simulink model "SAC_simulink"  (R2025b)
settings: Solver=ode4  StartTime=0.0  StopTime=180  FixedStep=0.01  RelTol=1e-3
values from neighbouring files (symbols this model uses):
  action_limits_lower = 0.88    [main_SAC.m]
  action_limits_upper = 1.07    [main_SAC.m]
  b0 = (1-t)^3    [ph7_teta_vincolato_new.m]
  k = Num_k./(Den_k + 1e-6)    [ph7_teta_vincolato_new.m]
  par_phys = struct    [main_SAC.m]    (also in test_all_agents_random_training_domain.m)
  rigeneration_step_s = 300    [main_SAC.m]
  T = resultsTable(ok, :)    [test_all_agents_random_training_domain.m]
  target = [0; 0; 0]    [test_all_agents_random_training_domain.m]
  Ts = 150    [main_SAC.m]    (also in test_all_agents_random_training_domain.m)
undefined symbols (not defined in the file or in its folder): delay, delta_a_max, h_max, h_min, k0_target, k1_target, k_L, max_idx, mean_vertical_velocity, meters_end_zf, r_max, r_min, s_f_time, t1_max_rad, t1_min_rad, t_step, wc, X0, yaw_max, yaw_min
libraries: slctrl_adaptive x3, aerolibobsolete x1, aerolibasang x1, simulink x1, aerolibatmos2 x1, rllib x1
(part 1 of 2)
settings Model: PauseTimes=0.01  PacingRate=0.200000  Creator=massy  LastModifiedBy=nicom
settings DebuggingCC: UnconnectedInputMsg=warning  UnconnectedOutputMsg=warning  UnconnectedLineMsg=warning
settings ModelReferenceCC: EnableRefExpFcnMdlSchedulingChecks=on
settings RTWCC: GPUComputeCapability=3.5  DLArmComputeVersion=19.05

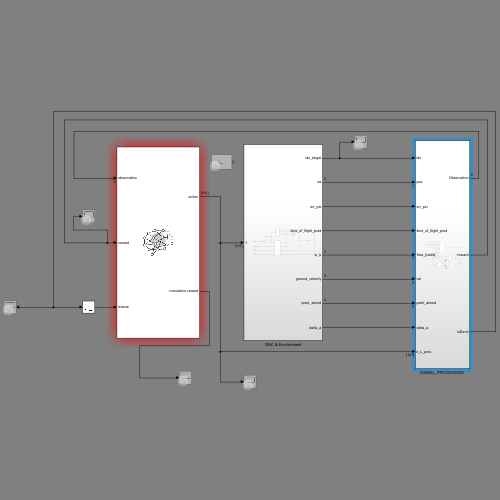
[thumbnail: Simulink's stored preview of the top-level diagram]
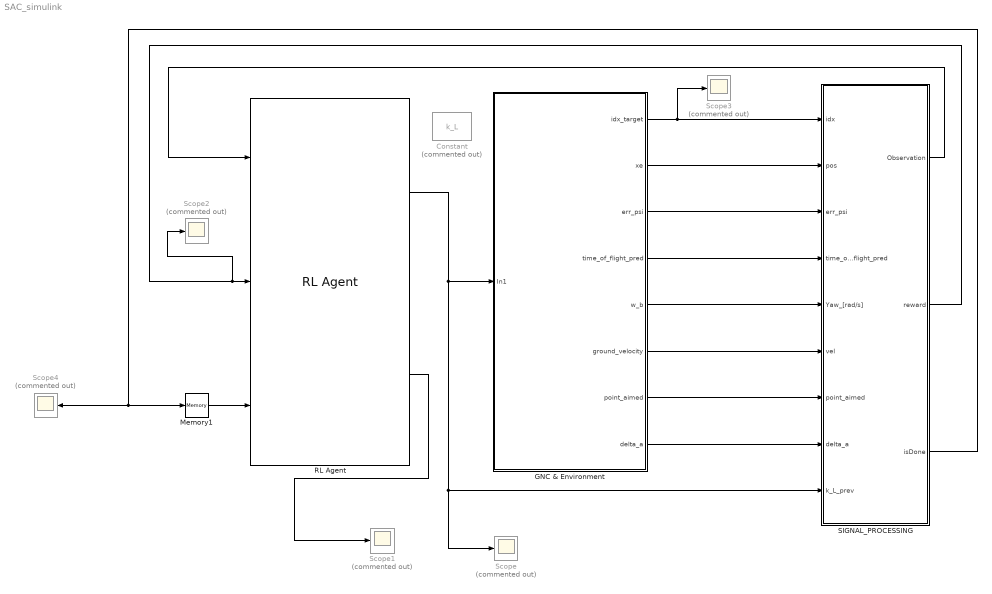
== system SAC_simulink ==
  Constant : Constant  Commented=on  Value=k_L
  GNC & Environment : Subsystem
  Memory1 : Memory
  RL Agent : rllib/RL Agent  Agent=agent  ExternalActionAsInput=off  ProvideLastAction=off  ProvideCumRwd=on  TreatAsDirectFeedthrough=on  UseStrictObservationDataTypes=off
  "SIGNAL_PROCESSING " : Subsystem
  Scope{,1..4} (5 alike) : Scope  Commented=on
      Scope settings: ActiveDisplayYMinimum=0.48959660530090332  ActiveDisplayYMaximum=2.4895966053009033  DataLoggingVariableName=ScopeData29
      Scope1 settings: ActiveDisplayYMinimum=-18280.567213697534  ActiveDisplayYMaximum=2455.6337548888514  DataLoggingVariableName=ScopeData35
      Scope2 settings: ActiveDisplayYMinimum=-16245.428943711315  ActiveDisplayYMaximum=-3791.1395065981656  DataLoggingVariableName=ScopeData36
      Scope3 settings: ActiveDisplayYMinimum=-22.849241680887388  ActiveDisplayYMaximum=119.97274269411264  DataLoggingVariableName=ScopeData37
      Scope4 settings: ActiveDisplayYMinimum=-0.12499999999999997  ActiveDisplayYMaximum=1.125  DataLoggingVariableName=ScopeData14
  wires:
  "SIGNAL_PROCESSING "/1(Observation) -> RL Agent/1
  GNC & Environment/1(idx_target) -> Scope3/1, "SIGNAL_PROCESSING "/1(idx)
  GNC & Environment/3(err_psi) -> "SIGNAL_PROCESSING "/3(err_psi)
  GNC & Environment/2(xe) -> "SIGNAL_PROCESSING "/2(pos)
  Memory1/1 -> RL Agent/3
  RL Agent/1 -> Scope/1, "SIGNAL_PROCESSING "/9(k_L_prev), GNC & Environment/1(In1)
  GNC & Environment/8(delta_a) -> "SIGNAL_PROCESSING "/8(delta_a)
  GNC & Environment/6(ground_velocity) -> "SIGNAL_PROCESSING "/6(vel)
  GNC & Environment/4(time_of_flight_pred) -> "SIGNAL_PROCESSING "/4(time_of_flight_pred)
  GNC & Environment/7(point_aimed) -> "SIGNAL_PROCESSING "/7(point_aimed)
  GNC & Environment/5(w_b) -> "SIGNAL_PROCESSING "/5(Yaw_[rad/s])
  "SIGNAL_PROCESSING "/3(isDone) -> Scope4/1, Memory1/1
  RL Agent/2 -> Scope1/1
  "SIGNAL_PROCESSING "/2(reward) -> Scope2/1, RL Agent/2

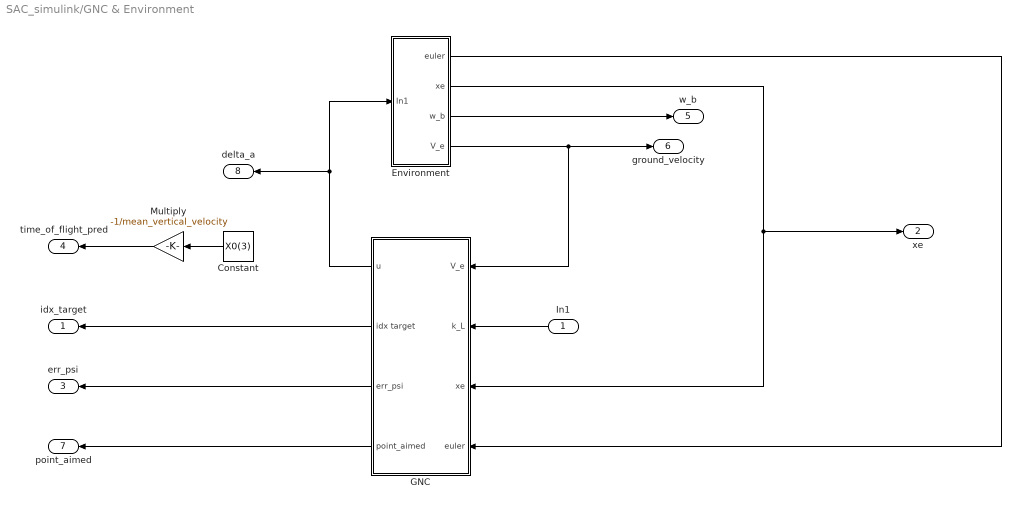
== system SAC_simulink/GNC & Environment ==
  In1 : Inport
  Constant : Constant  Value=X0(3)
  Environment : Subsystem
  GNC : Subsystem
  Multiply : Gain  Gain=-1/mean_vertical_velocity
  idx_target : Outport
  xe : Outport  Port=2
  err_psi : Outport  Port=3
  time_of_flight_pred : Outport  Port=4
  w_b : Outport  Port=5
  ground_velocity : Outport  Port=6
  point_aimed : Outport  Port=7
  delta_a : Outport  Port=8
  wires:
  Multiply/1 -> time_of_flight_pred/1
  GNC/3(err_psi) -> err_psi/1
  Environment/3(w_b) -> w_b/1
  Environment/1(euler) -> GNC/4(euler)
  Environment/2(xe) -> GNC/3(xe), xe/1
  GNC/2(idx target) -> idx_target/1
  GNC/1(u) -> delta_a/1, Environment/1(In1)
  Environment/4(V_e) -> ground_velocity/1, GNC/1(V_e)
  GNC/4(point_aimed) -> point_aimed/1
  Constant/1 -> Multiply/1
  In1/1 -> GNC/2(k_L)

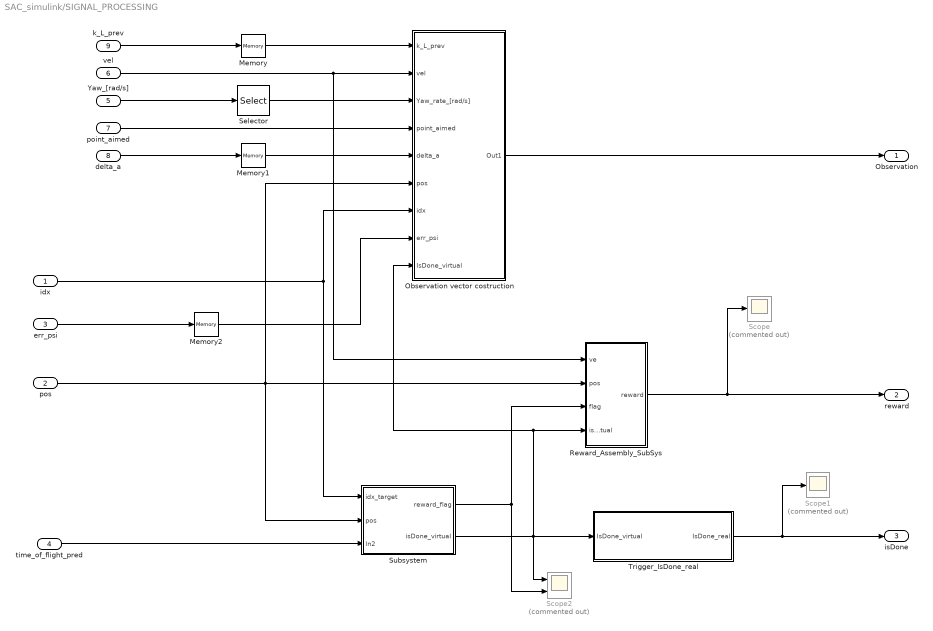
== system SAC_simulink/SIGNAL_PROCESSING  ==
  idx : Inport
  pos : Inport  Port=2
  err_psi : Inport  Port=3
  time_of_flight_pred : Inport  Port=4
  Yaw_[rad/s] : Inport  Port=5
  vel : Inport  Port=6
  point_aimed : Inport  Port=7
  delta_a : Inport  Port=8
  k_L_prev : Inport  Port=9
  Memory : Memory
  Memory1 : Memory
  Memory2 : Memory
  Observation vector costruction : Subsystem
  Reward_Assembly_SubSys : Subsystem
  Scope : Scope  Commented=on
      settings: ActiveDisplayYMinimum=-21750  ActiveDisplayYMaximum=-14250
  Scope1 : Scope  Commented=on
      settings: ActiveDisplayYMinimum=-0.72691328594836357  ActiveDisplayYMaximum=2.2813607561654949  DataLoggingVariableName=ScopeData17
  Scope2 : Scope  Commented=on  NumInputPorts=2
      settings: ActiveDisplayYMinimum=-0.13410064239828712  ActiveDisplayYMaximum=1.3815578158458244  DataLoggingVariableName=ScopeData18
  Selector : Selector  InputPortWidth=3  IndexOptions=Index vector (dialog)  Indices=[ 3]  OutputSizes=1
  Subsystem : Subsystem
  Trigger_IsDone_real : Subsystem
  Observation : Outport
  reward : Outport  Port=2
  isDone : Outport  Port=3
  wires:
  Subsystem/1(reward_flag) -> Scope2/2, Reward_Assembly_SubSys/3(flag)
  idx/1 -> Observation vector costruction/7(idx), Subsystem/1(idx_target)
  err_psi/1 -> Memory2/1
  point_aimed/1 -> Observation vector costruction/4(point_aimed)
  Subsystem/2(isDone_virtual) -> Scope2/1, Trigger_IsDone_real/1(IsDone_virtual), Reward_Assembly_SubSys/4(isDone_virtual), Observation vector costruction/9(IsDone_virtual)
  pos/1 -> Subsystem/2(pos), Reward_Assembly_SubSys/2(pos), Observation vector costruction/6(pos)
  Reward_Assembly_SubSys/1(reward) -> Scope/1, reward/1
  Yaw_[rad/s]/1 -> Selector/1
  time_of_flight_pred/1 -> Subsystem/3(In2)
  Observation vector costruction/1(Out1) -> Observation/1
  delta_a/1 -> Memory1/1
  Selector/1 -> Observation vector costruction/3(Yaw_rate_[rad/s])
  Trigger_IsDone_real/1(IsDone_real) -> Scope1/1, isDone/1
  k_L_prev/1 -> Memory/1
  vel/1 -> Reward_Assembly_SubSys/1(ve), Observation vector costruction/2(vel)
  Memory1/1 -> Observation vector costruction/5(delta_a)
  Memory2/1 -> Observation vector costruction/8(err_psi)
  Memory/1 -> Observation vector costruction/1(k_L_prev)

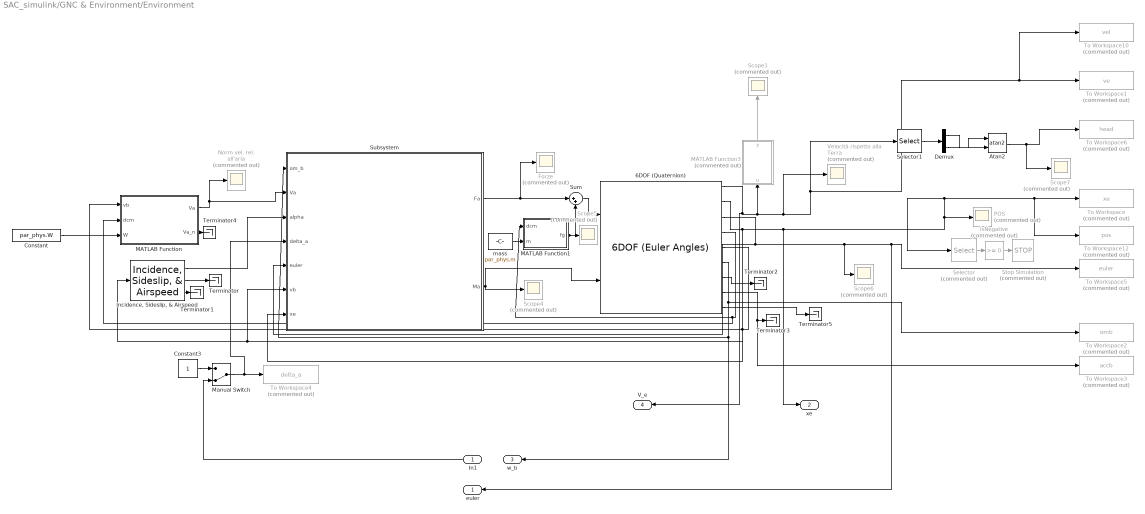
== system SAC_simulink/GNC & Environment/Environment ==
  In1 : Inport
  6DOF (Quaternion) : aerolibobsolete/6DOF (Euler Angles)  units=Metric (MKS)  mtype=Fixed  rep=Quaternion  xme_0=X0  Vm_0=V0  eul_0=euler  pm_0=w0  mass_0=par_phys.m  mass_e=0.5  mass_f=2.0  inertia=par_phys.I  inertia_e=eye(3)  inertia_f=2*eye(3)  k_quat=1.0  vre_flag=on  abi_flag=on  aMode=0  xme_statename=''  Vm_statename=''  eul_statename=''  quat_statename=''  pm_statename=''  mass_statename=''
  Atan2 : Trigonometry  Operator=atan2
  Constant : Constant  Value=par_phys.W
  Constant3 : Constant
  Demux : Demux  Outputs=2
  Forze : Scope  Commented=on
      settings: ActiveDisplayYMinimum=-111.7562  ActiveDisplayYMaximum=149.47198  DataLoggingVariableName=ScopeData4
  "Incidence, Sideslip, & Airspeed" : aerolibasang/Incidence, Sideslip, & Airspeed
  IsNegative : simulink/Logic and Bit Operations/Compare To Zero  Commented=on  relop=>=  OutDataTypeStr=boolean
      settings: LibrarySourceBlock=|
      | simulink/Quick Insert/Logic and Bit
      | Operations/IsNegative
  MATLAB Function : MATLAB Function  TreatAsAtomicUnit=on
  MATLAB Function1 : MATLAB Function  TreatAsAtomicUnit=on
  MATLAB Function3 : MATLAB Function  Commented=on  TreatAsAtomicUnit=on
  Manual Switch : ManualSwitch  CurrentSetting=0
  Norm vel. rel. all'aria : Scope  Commented=on
      settings: ActiveDisplayYMinimum=8.90491  ActiveDisplayYMaximum=12.9997  DataLoggingVariableName=ScopeData3
  POS : Scope  Commented=on
      settings: ActiveDisplayYMinimum=-1583.3551657510689  ActiveDisplayYMaximum=8026.0269716415532
  Scope{1,4..7} (5 alike) : Scope  Commented=on
      Scope1 settings: ActiveDisplayYMinimum=-1  ActiveDisplayYMaximum=1
      Scope4 settings: ActiveDisplayYMinimum=-1.26764  ActiveDisplayYMaximum=1.42182  DataLoggingVariableName=ScopeData5
      Scope5 settings: ActiveDisplayYMinimum=-38.15496  ActiveDisplayYMaximum=51.10944  DataLoggingVariableName=ScopeData6
      Scope6 settings: ActiveDisplayYMinimum=-1  ActiveDisplayYMaximum=1
      Scope7 settings: ActiveDisplayYMinimum=-1  ActiveDisplayYMaximum=1
  Selector : Selector  Commented=on  InputPortWidth=3  IndexOptions=Index vector (dialog)  Indices=[3]  OutputSizes=1
  Selector1 : Selector  InputPortWidth=3  IndexOptions=Index vector (dialog)  Indices=[1 2]  OutputSizes=1
  Stop Simulation : Stop  Commented=on
  Subsystem : Subsystem
  Sum : Sum  Inputs=|++
  Terminator{,1..5} (6 alike) : Terminator
  To Workspace : ToWorkspace  Commented=on  VariableName=xe  SampleTime=-1
  To Workspace1 : ToWorkspace  Commented=on  VariableName=ve  SampleTime=-1
  To Workspace10 : ToWorkspace  Commented=on  VariableName=vel  SaveFormat=Timeseries  SampleTime=-1
  To Workspace12 : ToWorkspace  Commented=on  VariableName=pos  SaveFormat=Timeseries  SampleTime=-1
  To Workspace2 : ToWorkspace  Commented=on  VariableName=omb  SampleTime=-1
  To Workspace3 : ToWorkspace  Commented=on  VariableName=accb  SampleTime=-1
  To Workspace4 : ToWorkspace  Commented=on  VariableName=delta_a  SampleTime=-1
  To Workspace5 : ToWorkspace  Commented=on  VariableName=euler  SampleTime=-1
  To Workspace6 : ToWorkspace  Commented=on  VariableName=head  SampleTime=-1
  Velocità rispetto alla Terra : Scope  Commented=on
      settings: ActiveDisplayYMinimum=-13.738515568500244  ActiveDisplayYMaximum=14.244609911524053  DataLoggingVariableName=ScopeData2
  mass : Constant  Value=par_phys.m
  euler : Outport
  xe : Outport  Port=2
  w_b : Outport  Port=3
  V_e : Outport  Port=4
  wires:
  Constant/1 -> MATLAB Function/3(W)
  Subsystem/2(Ma) -> Scope4/1, 6DOF (Quaternion)/2
  MATLAB Function1/1(fg) -> Sum/2, Scope5/1
  MATLAB Function/1(Va) -> Norm vel. rel. all'aria/1, Subsystem/2(Va)
  Constant3/1 -> Manual Switch/1
  6DOF (Quaternion)/3 -> Subsystem/5(euler), euler/1, To Workspace5/1, Scope6/1
  Atan2/1 -> Scope7/1, To Workspace6/1
  6DOF (Quaternion)/7 -> Terminator2/1
  Selector1/1 -> Demux/1
  Subsystem/1(Fa) -> Forze/1, Sum/1
  6DOF (Quaternion)/6 -> To Workspace2/1, w_b/1, Subsystem/1(om_b)
  MATLAB Function3/1(y) -> Scope1/1
  6DOF (Quaternion)/2 -> xe/1, Selector/1, To Workspace12/1, To Workspace/1, POS/1, Subsystem/7(xe)
  6DOF (Quaternion)/4 -> MATLAB Function1/1(dcm), MATLAB Function/2(dcm)
  6DOF (Quaternion)/5 -> "Incidence, Sideslip, & Airspeed"/1, Subsystem/6(vb), MATLAB Function/1(vb)
  In1/1 -> Manual Switch/2
  6DOF (Quaternion)/8 -> To Workspace3/1, Terminator3/1
  "Incidence, Sideslip, & Airspeed"/2 -> Terminator/1
  Sum/1 -> 6DOF (Quaternion)/1
  Demux/2 -> Atan2/1
  Demux/1 -> Atan2/2
  "Incidence, Sideslip, & Airspeed"/1 -> Subsystem/3(alpha)
  "Incidence, Sideslip, & Airspeed"/3 -> Terminator1/1
  Manual Switch/1 -> Subsystem/4(delta_a), To Workspace4/1
  mass/1 -> MATLAB Function1/2(m)
  MATLAB Function/2(Va_n) -> Terminator4/1
  6DOF (Quaternion)/1 -> V_e/1, Selector1/1, To Workspace10/1, To Workspace1/1, Velocità rispetto alla Terra/1, MATLAB Function3/1(u)
  Selector/1 -> IsNegative/1
  IsNegative/1 -> Stop Simulation/1
  6DOF (Quaternion)/9 -> Terminator5/1

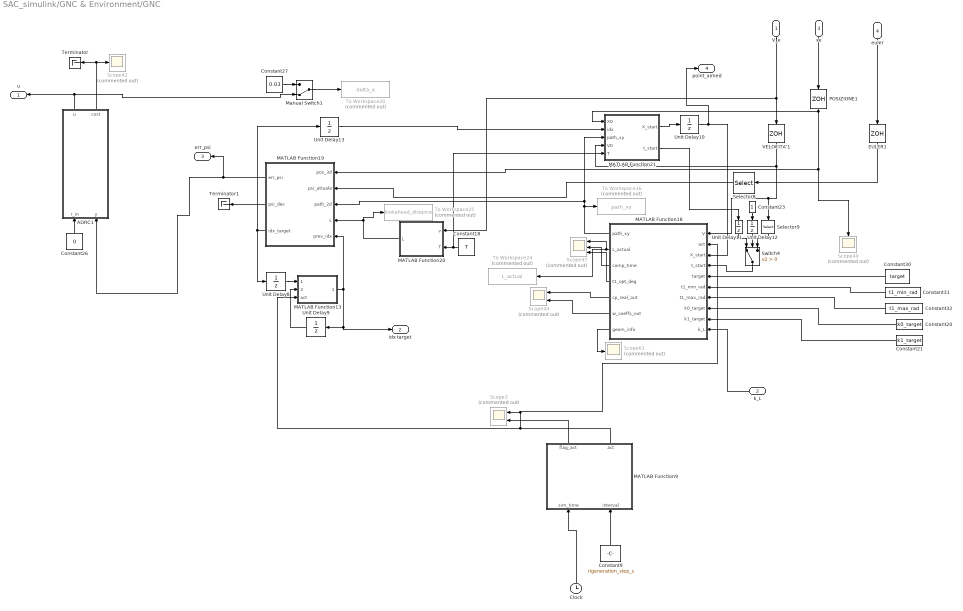
== system SAC_simulink/GNC & Environment/GNC ==
  V_e : Inport
  k_L : Inport  Port=2
  xe : Inport  Port=3
  euler : Inport  Port=4
  ADRC1 : Subsystem  mask{b0=-b0, wc=wc, wo=k*wc, Ts=t_step, x0=0, sat_u=0.03, sat_l=-0.03, rate_u=0.006, rate_l=-0.006}
      mask prompts: b0 "Critical Gain b0"; wc "Controller Bandwidth (rad/sec)"; wo "Observer Bandwidth (rad/sec)"; Ts "Sample Time"; x0 "Initial Condition"; sat_u "Upper bound"; sat_l "Lower bound"; rate_u "Upper bound"; rate_l "Lower bound"
      mask init:
      | % --- Codice di Inizializzazione Maschera ADRC ---
      | 
      | % 1. Calcolo dei parametri ESO
      | % (Mappa la bandwidth 'wo' nel dominio discreto Z)
      | beta = exp(-wo * Ts);
      | 
      | % 2. Guadagni Luenberger (vettore L)
      | % Formule per posizionare i 3 poli dell'osservatore in 'beta'
      | l1 = 1 - beta^3;
      | l2 = (3*(1-beta)^2 * (1+beta)) / (2*Ts);
      | l3 = (1-beta)^3 / (Ts^2);
      | 
      | % Vettore che i Gain interni si aspettano
      | ld = [l1; l2; l3]; 
      | 
      | % 3. Matrice Sistema Discreto (Ad)
      | % Modello doppio integratore (posizione, velocità, disturbo)
      | ad = [1, Ts, Ts^2/2;
      |       0,  1,    Ts;
      |       0,  0,     1];
      | 
      | % 4. Matrice Ingresso Discreto (Bd)
      | bd = [b0 * Ts^2/2;
      |       b0 * Ts;
      |       0];
      | 
      | % 5. Matrice Uscita (C)
      | c = [1 0 0];
      mask DialogControl DescTextVar Prompt: Parameters ADRC
      mask DialogControl Saturation Prompt: Saturation
      mask DialogControl Container4 Prompt: Rate Limiter
  Clock : Clock
  Constant18 : Constant  Value=T
  Constant20 : Constant  Value=k0_target
  Constant21 : Constant  Value=k1_target
  Constant23 : Constant
  Constant26 : Constant  Value=0
  Constant27 : Constant  Value=0.03
  Constant30 : Constant  Value=target
  Constant31 : Constant  Value=t1_min_rad
  Constant32 : Constant  Value=t1_max_rad
  Constant9 : Constant  Value=rigeneration_step_s
  EULER1 : ZeroOrderHold  SampleTime=-1
  MATLAB Function13 : MATLAB Function  TreatAsAtomicUnit=on
  MATLAB Function18 : MATLAB Function  TreatAsAtomicUnit=on
  MATLAB Function19 : MATLAB Function  TreatAsAtomicUnit=on
  MATLAB Function20 : MATLAB Function  TreatAsAtomicUnit=on
  MATLAB Function21 : MATLAB Function  TreatAsAtomicUnit=on
  MATLAB Function9 : MATLAB Function  TreatAsAtomicUnit=on
  Manual Switch1 : ManualSwitch  CurrentSetting=0
  POSIZIONE1 : ZeroOrderHold  SampleTime=-1
  Scope3 : Scope  Commented=on  NumInputPorts=2
      settings: ActiveDisplayYMinimum=-1.25  ActiveDisplayYMaximum=1.25  DataLoggingVariableName=ScopeData8
  Scope40 : Scope  Commented=on
      settings: ActiveDisplayYMinimum=-341.60221967749681  ActiveDisplayYMaximum=750.13712237085417  DataLoggingVariableName=ScopeData73
  Scope42 : Scope  Commented=on
      settings: ActiveDisplayYMinimum=-1  ActiveDisplayYMaximum=1  DataLoggingVariableName=ScopeData75
  Scope44 : Scope  Commented=on  NumInputPorts=2
      settings: ActiveDisplayYMinimum=-745.73859428255776  ActiveDisplayYMaximum=1354.574191363215  DataLoggingVariableName=ScopeData77
  Scope47 : Scope  Commented=on  NumInputPorts=3
      settings: ActiveDisplayYMinimum=-1672.2830379019078  ActiveDisplayYMaximum=3185.7011907738192  DataLoggingVariableName=ScopeData80
  Scope61 : Scope  Commented=on
      settings: DataLoggingVariableName=ScopeData94
  Selector8 : Selector  InputPortWidth=3  IndexOptions=Index vector (dialog)  Indices=3  OutputSizes=1
  Selector9 : Selector  InputPortWidth=3  IndexOptions=Index vector (dialog)  Indices=[1 2]  OutputSizes=1
  Switch4 : Switch  Criteria=u2 > Threshold  SaturateOnIntegerOverflow=off  InputSameDT=off
  Terminator : Terminator
  Terminator1 : Terminator
  To Workspace16 : ToWorkspace  Commented=on  VariableName=path_xy  SaveFormat=Timeseries  SampleTime=-1
  To Workspace20 : ToWorkspace  Commented=on  VariableName=delta_a  SampleTime=-1
  To Workspace24 : ToWorkspace  Commented=on  VariableName=L_actual  SaveFormat=Timeseries  SampleTime=-1
  To Workspace25 : ToWorkspace  Commented=on  VariableName=lookahead_distance  SaveFormat=Timeseries  SampleTime=-1
  Unit Delay10 : UnitDelay  InitialCondition=X0  SampleTime=-1  HasFrameUpgradeWarning=on
  Unit Delay11 : UnitDelay  InitialCondition=[0;0]  SampleTime=-1  HasFrameUpgradeWarning=on
  Unit Delay12 : UnitDelay  InitialCondition=[0;0]  SampleTime=-1  HasFrameUpgradeWarning=on
  Unit Delay13 : UnitDelay  InitialCondition=1  SampleTime=-1  HasFrameUpgradeWarning=on
  Unit Delay8 : UnitDelay  InitialCondition=1  SampleTime=-1  HasFrameUpgradeWarning=on
  Unit Delay9 : UnitDelay  InitialCondition=1  SampleTime=-1  HasFrameUpgradeWarning=on
  VELOCITA'1 : ZeroOrderHold  SampleTime=-1
  u : Outport
  idx target : Outport  Port=2
  err_psi : Outport  Port=3
  point_aimed : Outport  Port=4
  wires:
  MATLAB Function18/7(geom_info) -> Scope61/1
  Unit Delay8/1 -> MATLAB Function13/1(prev_idx)
  MATLAB Function18/2(L_actual) -> To Workspace24/1, Scope47/1
  MATLAB Function18/6(w_coeffs_out) -> Scope44/2
  Constant27/1 -> Manual Switch1/1
  Switch4/1 -> MATLAB Function18/4(t_start)
  MATLAB Function20/1(L) -> To Workspace25/1, MATLAB Function19/4(L)
  Unit Delay12/1 -> Switch4/2
  Manual Switch1/1 -> To Workspace20/1
  MATLAB Function21/1(X_start) -> Unit Delay10/1
  Unit Delay13/1 -> MATLAB Function21/2(idx)
  MATLAB Function18/1(path_xy) -> To Workspace16/1, MATLAB Function21/3(path_xy), MATLAB Function19/3(path_2d)
  Selector9/1 -> Switch4/3
  Constant20/1 -> MATLAB Function18/8(k0_target)
  Constant31/1 -> MATLAB Function18/6(t1_min_rad)
  MATLAB Function18/4(t1_opt_deg) -> Scope47/3
  MATLAB Function21/2(t_start) -> Unit Delay11/1
  Constant21/1 -> MATLAB Function18/9(k1_target)
  Constant26/1 -> ADRC1/1(r_in)
  POSIZIONE1/1 -> Scope40/1, MATLAB Function19/1(pos_3d), MATLAB Function21/1(X0)
  MATLAB Function19/1(err_psi) -> ADRC1/2(y), err_psi/1
  Unit Delay9/1 -> MATLAB Function13/2(old_idx)
  Unit Delay11/1 -> Switch4/1
  Constant32/1 -> MATLAB Function18/7(t1_max_rad)
  MATLAB Function13/1(prev_idx_clean) -> idx target/1, Unit Delay9/1, MATLAB Function19/5(prev_idx)
  MATLAB Function19/3(idx_target) -> Unit Delay13/1, Unit Delay8/1
  MATLAB Function18/3(comp_time) -> Scope47/2
  MATLAB Function18/5(cp_real_out) -> Scope44/1
  Constant23/1 -> Unit Delay12/1
  ADRC1/2(cost) -> Terminator/1, Scope42/1
  Selector8/1 -> MATLAB Function19/2(psi_attuale)
  EULER1/1 -> Selector8/1
  VELOCITA'1/1 -> MATLAB Function18/1(V), Selector9/1, MATLAB Function21/4(V0)
  Constant18/1 -> MATLAB Function21/5(T), MATLAB Function20/2(T)
  Constant30/1 -> MATLAB Function18/5(target)
  Unit Delay10/1 -> point_aimed/1, MATLAB Function18/3(X_start)
  ADRC1/1(u) -> Manual Switch1/2, u/1
  k_L/1 -> MATLAB Function18/10(k_L)
  euler/1 -> EULER1/1
  xe/1 -> POSIZIONE1/1
  V_e/1 -> VELOCITA'1/1, MATLAB Function20/1(v)
  MATLAB Function9/2(act) -> MATLAB Function13/3(act), MATLAB Function18/2(act), Scope3/1
  Clock/1 -> MATLAB Function9/1(sim_time)
  MATLAB Function9/1(flag_act) -> Scope3/2
  Constant9/1 -> MATLAB Function9/2(interval)
  MATLAB Function19/2(psi_des) -> Terminator1/1

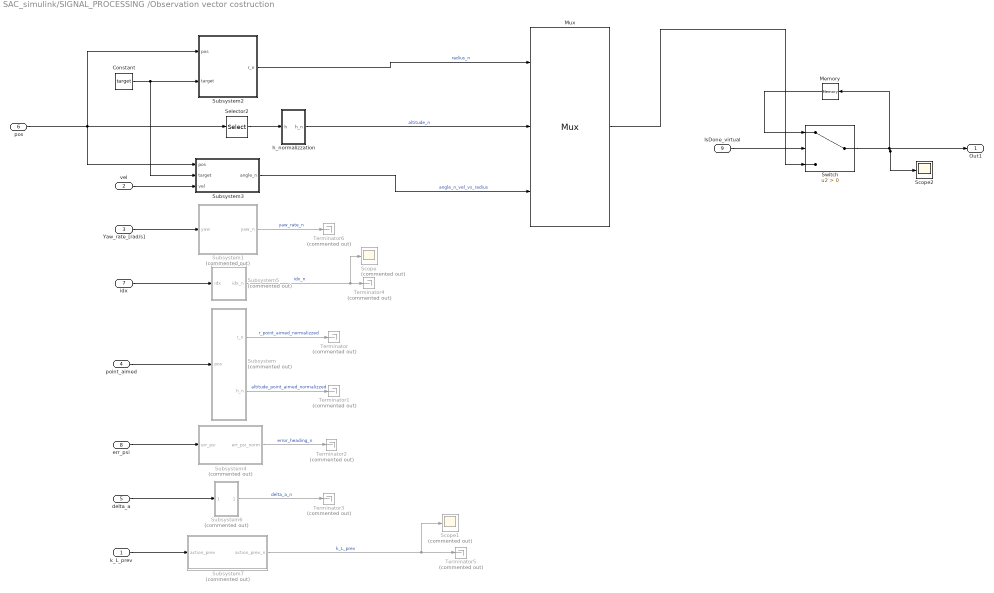
== system SAC_simulink/SIGNAL_PROCESSING /Observation vector costruction ==
  k_L_prev : Inport
  vel : Inport  Port=2
  Yaw_rate_[rad/s] : Inport  Port=3
  point_aimed : Inport  Port=4
  delta_a : Inport  Port=5
  pos : Inport  Port=6
  idx : Inport  Port=7
  err_psi : Inport  Port=8
  IsDone_virtual : Inport  Port=9
  Constant : Constant  Value=target
  Memory : Memory
  Mux : Mux  Inputs=3
  Scope : Scope  Commented=on
      settings: ActiveDisplayYMinimum=-1  ActiveDisplayYMaximum=1  DataLoggingVariableName=ScopeData15
  Scope1 : Scope  Commented=on
      settings: ActiveDisplayYMinimum=-0.23571507632732391  ActiveDisplayYMaximum=0.58297414848437679  DataLoggingVariableName=ScopeData23
  Scope2 : Scope
      settings: ActiveDisplayYMinimum=-1.1917806646843343  ActiveDisplayYMaximum=0.84683416251059906  DataLoggingVariableName=ScopeData25
  Selector2 : Selector  InputPortWidth=3  IndexOptions=Index vector (dialog)  Indices=[3]  OutputSizes=1
  Subsystem : Subsystem  Commented=on
  Subsystem1 : Subsystem  Commented=on
  Subsystem2 : Subsystem
  Subsystem3 : Subsystem
  Subsystem4 : Subsystem  Commented=on
  Subsystem5 : Subsystem  Commented=on
  Subsystem6 : Subsystem  Commented=on
  Subsystem7 : Subsystem  Commented=on
  Switch : Switch  Criteria=u2 > Threshold  SaturateOnIntegerOverflow=off  InputSameDT=off
  Terminator{,1..6} (7 alike) : Terminator  Commented=on
  h_normalizzation : Subsystem
  Out1 : Outport
  wires:
  Constant/1 -> Subsystem3/2(target), Subsystem2/2(target)
  Mux/1 -> Switch/3
  pos/1 -> Subsystem2/1(pos), Selector2/1, Subsystem3/1(pos)
  Selector2/1 -> h_normalizzation/1(h)
  h_normalizzation/1(h_n) -> Mux/2  "altitude_n"
  point_aimed/1 -> Subsystem/1(pos)
  Subsystem/1(r_n) -> Terminator/1  "r_point_aimed_normalizzed"
  Subsystem/2(h_n) -> Terminator1/1  "altitude_point_aimed_normalizzed"
  Yaw_rate_[rad/s]/1 -> Subsystem1/1(yaw)
  Subsystem1/1(yaw_n) -> Terminator6/1  "yaw_rate_n"
  Subsystem2/1(r_n) -> Mux/1  "radius_n"
  vel/1 -> Subsystem3/3(vel)
  Subsystem3/1(angle_n) -> Mux/3  "angle_n_vel_vs_radius"
  err_psi/1 -> Subsystem4/1(err_psi)
  Subsystem4/1(err_psi_norm) -> Terminator2/1  "error_heading_n"
  idx/1 -> Subsystem5/1(idx)
  Subsystem5/1(idx_n) -> Terminator4/1, Scope/1  "idx_n"
  delta_a/1 -> Subsystem6/1(In1)
  Subsystem6/1(Out1) -> Terminator3/1  "delta_a_n"
  k_L_prev/1 -> Subsystem7/1(action_prev)
  Subsystem7/1(action_prev_n) -> Terminator5/1, Scope1/1  "k_L_prev"
  IsDone_virtual/1 -> Switch/2
  Switch/1 -> Scope2/1, Out1/1, Memory/1
  Memory/1 -> Switch/1

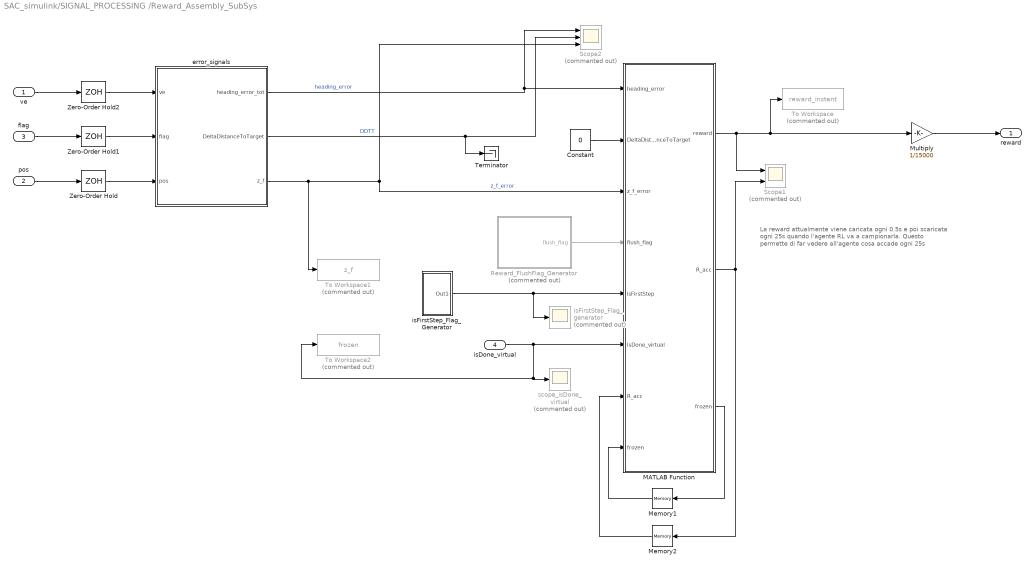
== system SAC_simulink/SIGNAL_PROCESSING /Reward_Assembly_SubSys ==
  note: La reward attualmente viene caricata ogni 0.5s e poi scaricata ogni 25s quando l'agente RL va a campionarla. Questo permette di far vedere all'agente cosa accade ogni 25s
  ve : Inport
  pos : Inport  Port=2
  flag : Inport  Port=3
  isDone_virtual : Inport  Port=4
  Constant : Constant  Value=0
  MATLAB Function : MATLAB Function  TreatAsAtomicUnit=on
  Memory1 : Memory
  Memory2 : Memory  InitialCondition=-15000
  Multiply : Gain  Gain=1/15000
  Reward_FlushFlag_Generator : Subsystem  Commented=on
  Scope1 : Scope  Commented=on  NumInputPorts=2
      settings: ActiveDisplayYMinimum=-21750  ActiveDisplayYMaximum=-14250  DataLoggingVariableName=ScopeData10
  Scope2 : Scope  Commented=on  NumInputPorts=3
      settings: ActiveDisplayYMinimum=-8459.6713424506361  ActiveDisplayYMaximum=2093.5818274712415  DataLoggingVariableName=ScopeData9
  Terminator : Terminator
  To Workspace : ToWorkspace  Commented=on  VariableName=reward_instant  SaveFormat=Timeseries  SampleTime=-1
  To Workspace1 : ToWorkspace  Commented=on  VariableName=z_f  SaveFormat=Timeseries  SampleTime=-1
  To Workspace2 : ToWorkspace  Commented=on  VariableName=frozen  SaveFormat=Timeseries  SampleTime=-1
  Zero-Order Hold : ZeroOrderHold  SampleTime=-1
  Zero-Order Hold1 : ZeroOrderHold  SampleTime=-1
  Zero-Order Hold2 : ZeroOrderHold  SampleTime=-1
  error_signals : Subsystem
  isFirstStep_Flag_Generator : Subsystem
  isFirstStep_Flag_generator : Scope  Commented=on
      settings: ActiveDisplayYMinimum=-0.12499999999999997  ActiveDisplayYMaximum=1.125  DataLoggingVariableName=ScopeData21
  scope_isDone_virtual : Scope  Commented=on
      settings: ActiveDisplayYMinimum=-0.12499999999999997  ActiveDisplayYMaximum=1.125  DataLoggingVariableName=ScopeData30
  reward : Outport
  wires:
  error_signals/3(z_f) -> MATLAB Function/3(z_f_error), Scope2/3, To Workspace1/1  "z_f_error"
  error_signals/2(DeltaDistanceToTarget) -> Terminator/1, Scope2/2  "DDTT"
  ve/1 -> Zero-Order Hold2/1
  flag/1 -> Zero-Order Hold1/1
  pos/1 -> Zero-Order Hold/1
  MATLAB Function/1(reward) -> Scope1/1, To Workspace/1, Multiply/1
  isDone_virtual/1 -> To Workspace2/1, scope_isDone_virtual/1, MATLAB Function/6(IsDone_virtual)
  MATLAB Function/3(frozen) -> Memory1/1
  MATLAB Function/2(R_acc) -> Memory2/1, Scope1/2
  error_signals/1(heading_error_tot) -> MATLAB Function/1(heading_error), Scope2/1  "heading_error"
  Reward_FlushFlag_Generator/1(flush_flag) -> MATLAB Function/4(flush_flag)
  Memory1/1 -> MATLAB Function/8("frozen ")
  Memory2/1 -> MATLAB Function/7("R_acc ")
  isFirstStep_Flag_Generator/1(Out1) -> isFirstStep_Flag_generator/1, MATLAB Function/5(isFirstStep)
  Constant/1 -> MATLAB Function/2(DeltaDistanceToTarget)
  Zero-Order Hold2/1 -> error_signals/1(ve)
  Zero-Order Hold1/1 -> error_signals/2(flag)
  Zero-Order Hold/1 -> error_signals/3(pos)
  Multiply/1 -> reward/1

== system SAC_simulink/SIGNAL_PROCESSING /Subsystem ==
  idx_target : Inport
  pos : Inport  Port=2
  In2 : Inport  Port=3
  FLAG CHOOSER : Subsystem
  Memory : Memory
  To Workspace8 : ToWorkspace  Commented=on  VariableName=reward_flag  SaveFormat=Timeseries  SampleTime=-1
      settings: MaxDataPoints=1
  To Workspace9 : ToWorkspace  Commented=on  VariableName=dt_pred  SaveFormat=Timeseries  SampleTime=-1
  reward_flag : Outport
  isDone_virtual : Outport  Port=2
  wires:
  Memory/1 -> FLAG CHOOSER/2(dt_flight), To Workspace9/1
  pos/1 -> FLAG CHOOSER/1(pos)
  FLAG CHOOSER/2(reward_flag) -> To Workspace8/1, reward_flag/1
  In2/1 -> Memory/1
  idx_target/1 -> FLAG CHOOSER/3(idx_target)
  FLAG CHOOSER/1(isDone_virtual) -> isDone_virtual/1

== system SAC_simulink/SIGNAL_PROCESSING /Trigger_IsDone_real ==
  IsDone_virtual : Inport
  Clock : Clock
  Constant : Constant  Value=Ts
  Constant1 : Constant  Value=t_step
  MATLAB Function : MATLAB Function  TreatAsAtomicUnit=on
  Memory : Memory
  Memory1 : Memory
  IsDone_real : Outport
  wires:
  Clock/1 -> MATLAB Function/1(t)
  IsDone_virtual/1 -> MATLAB Function/4(IsDone_virtual)
  Constant1/1 -> MATLAB Function/3(t_step)
  Constant/1 -> MATLAB Function/2(Ts)
  MATLAB Function/2(t_trigger) -> Memory/1
  MATLAB Function/3(armed) -> Memory1/1
  Memory/1 -> MATLAB Function/5("t_trigger ")
  Memory1/1 -> MATLAB Function/6("armed ")
  MATLAB Function/1(IsDone_real) -> IsDone_real/1

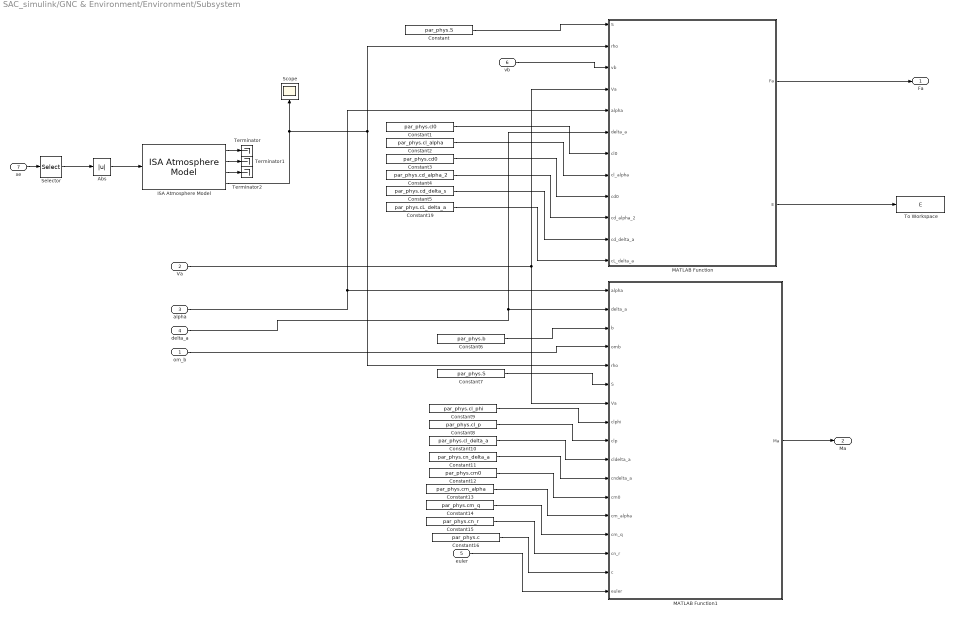
== system SAC_simulink/GNC & Environment/Environment/Subsystem ==
  om_b : Inport
  Va : Inport  Port=2
  alpha : Inport  Port=3
  delta_a : Inport  Port=4
  euler : Inport  Port=5
  vb : Inport  Port=6
  xe : Inport  Port=7
  Abs : Abs  SaturateOnIntegerOverflow=off
  Constant : Constant  Value=par_phys.S
  Constant1 : Constant  Value=par_phys.cl0
  Constant10 : Constant  Value=par_phys.cl_delta_a
  Constant11 : Constant  Value=par_phys.cn_delta_a
  Constant12 : Constant  Value=par_phys.cm0
  Constant13 : Constant  Value=par_phys.cm_alpha
  Constant14 : Constant  Value=par_phys.cm_q
  Constant15 : Constant  Value=par_phys.cn_r
  Constant16 : Constant  Value=par_phys.c
  Constant19 : Constant  Value=par_phys.cL_delta_a
  Constant2 : Constant  Value=par_phys.cl_alpha
  Constant3 : Constant  Value=par_phys.cd0
  Constant4 : Constant  Value=par_phys.cd_alpha_2
  Constant5 : Constant  Value=par_phys.cd_delta_s
  Constant6 : Constant  Value=par_phys.b
  Constant7 : Constant  Value=par_phys.S
  Constant8 : Constant  Value=par_phys.cl_p
  Constant9 : Constant  Value=par_phys.cl_phi
  ISA Atmosphere Model : aerolibatmos2/ISA Atmosphere Model  useExtended=off  action=None  custom=off  viscosityOut=off  g=9.80665  gamma=1.4  R=287.0531  L=0.0065  h_trop=11000  h_strat=20000  rho0=1.225  P0=101325  T0=288.15  h0=0  S=110.4  Tref=273.15  muref=1.716e-5
  MATLAB Function : MATLAB Function  TreatAsAtomicUnit=on
  MATLAB Function1 : MATLAB Function  TreatAsAtomicUnit=on
  Scope : Scope
      settings: ActiveDisplayYMinimum=0.38727  ActiveDisplayYMaximum=1.17808
  Selector : Selector  InputPortWidth=3  IndexOptions=Index vector (dialog)  Indices=[3]  OutputSizes=1
  Terminator : Terminator
  Terminator1 : Terminator
  Terminator2 : Terminator
  To Workspace : ToWorkspace  VariableName=E  SampleTime=-1
  Fa : Outport
  Ma : Outport  Port=2
  wires:
  Constant2/1 -> MATLAB Function/8(cl_alpha)
  Constant8/1 -> MATLAB Function1/9(clp)
  Constant10/1 -> MATLAB Function1/10(cldelta_a)
  Constant6/1 -> MATLAB Function1/3(b)
  Constant7/1 -> MATLAB Function1/6(S)
  Constant4/1 -> MATLAB Function/10(cd_alpha_2)
  Constant11/1 -> MATLAB Function1/11(cndelta_a)
  Constant15/1 -> MATLAB Function1/15(cn_r)
  Constant13/1 -> MATLAB Function1/13(cm_alpha)
  Constant14/1 -> MATLAB Function1/14(cm_q)
  Constant5/1 -> MATLAB Function/11(cd_delta_a)
  MATLAB Function1/1(Ma) -> Ma/1
  Constant1/1 -> MATLAB Function/7(cl0)
  Constant3/1 -> MATLAB Function/9(cd0)
  Constant9/1 -> MATLAB Function1/8(clphi)
  Constant/1 -> MATLAB Function/1(S)
  Constant16/1 -> MATLAB Function1/16(c)
  alpha/1 -> MATLAB Function/5(alpha), MATLAB Function1/1(alpha)
  Constant12/1 -> MATLAB Function1/12(cm0)
  om_b/1 -> MATLAB Function1/4(omb)
  delta_a/1 -> MATLAB Function/6(delta_a), MATLAB Function1/2(delta_a)
  MATLAB Function/1(Fa) -> Fa/1
  Va/1 -> MATLAB Function/4(Va), MATLAB Function1/7(Va)
  ISA Atmosphere Model/4 -> MATLAB Function1/5(rho), MATLAB Function/2(rho), Scope/1
  euler/1 -> MATLAB Function1/17(euler)
  Constant19/1 -> MATLAB Function/12(cL_delta_a)
  vb/1 -> MATLAB Function/3(vb)
  ISA Atmosphere Model/1 -> Terminator/1
  ISA Atmosphere Model/2 -> Terminator1/1
  ISA Atmosphere Model/3 -> Terminator2/1
  xe/1 -> Selector/1
  Selector/1 -> Abs/1
  Abs/1 -> ISA Atmosphere Model/1
  MATLAB Function/2(E) -> To Workspace/1

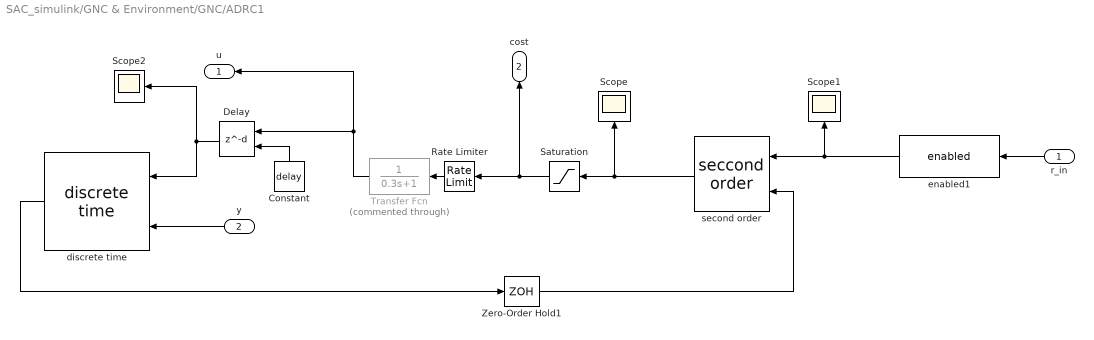
== system SAC_simulink/GNC & Environment/GNC/ADRC1 ==
  r_in : Inport
  y : Inport  Port=2
  Constant : Constant  Value=delay
  Delay : Delay  DelayLengthSource=Input port  DelayLength=50  DelayLengthUpperLimit=1000
      settings: InputPortMap=u0,p1
  Rate Limiter : RateLimiter  RisingSlewLimit=rate_u  FallingSlewLimit=rate_l
  Saturation : Saturate  UpperLimit=0.03  LowerLimit=-0.03
  Scope : Scope
      settings: ActiveDisplayYMinimum=-0.1062995848963169  ActiveDisplayYMaximum=0.029511302912964069  DataLoggingVariableName=ScopeData32
  Scope1 : Scope
      settings: ActiveDisplayYMinimum=0.831957554861144  ActiveDisplayYMaximum=1.2011935899740982  DataLoggingVariableName=ScopeData33
  Scope2 : Scope
      settings: ActiveDisplayYMinimum=-0.013678379699760226  ActiveDisplayYMaximum=-0.013594987250404263  DataLoggingVariableName=ScopeData34
  Transfer Fcn : TransferFcn  Commented=through  Denominator=[0.3 1]
  Zero-Order Hold1 : ZeroOrderHold  SampleTime=t_step
  discrete time : slctrl_adaptive/Active Disturbance Rejection Control/ADRC/extended state observer/discrete time  SystemSampleTime=-1  VariantControl=domain==2  VariantActivationTime=update diagram  EmptyChoice=off  PassThrough=off  PassThroughVariantControl=(default)  EmptyChoiceVariantControl=(default)  AllowFlexibleInterface=on  Latency=0  AutoFrameSizeCalculation=off
  enabled1 : slctrl_adaptive/Active Disturbance Rejection Control/ADRC/rZOH/enabled  SystemSampleTime=-1  VariantControl=domain==2  VariantActivationTime=update diagram  EmptyChoice=off  PassThrough=off  PassThroughVariantControl=(default)  EmptyChoiceVariantControl=(default)  AllowFlexibleInterface=on  Latency=0  AutoFrameSizeCalculation=off
  second order : slctrl_adaptive/Active Disturbance Rejection Control/ADRC/error feedback/seccond order  SystemSampleTime=-1  VariantControl=order ==2  VariantActivationTime=update diagram  EmptyChoice=off  PassThrough=off  PassThroughVariantControl=(default)  EmptyChoiceVariantControl=(default)  AllowFlexibleInterface=on  Latency=0  AutoFrameSizeCalculation=off
  u : Outport
  cost : Outport  Port=2
  wires:
  enabled1/1 -> second order/1, Scope1/1
  Saturation/1 -> Rate Limiter/1, cost/1
  r_in/1 -> enabled1/1
  Rate Limiter/1 -> Transfer Fcn/1
  y/1 -> discrete time/2
  second order/1 -> Saturation/1, Scope/1
  discrete time/1 -> Zero-Order Hold1/1
  Zero-Order Hold1/1 -> second order/2
  Transfer Fcn/1 -> Delay/1, u/1
  Delay/1 -> Scope2/1, discrete time/1
  Constant/1 -> Delay/2

== system SAC_simulink/SIGNAL_PROCESSING /Observation vector costruction/Subsystem ==
  pos : Inport
  Constant1 : Constant  Value=target
  Constant2 : Constant  Value=r_min
  Constant3 : Constant  Value=r_max
  Constant4 : Constant  Value=h_min
  Constant5 : Constant  Value=h_max
  MATLAB Function1 : MATLAB Function  TreatAsAtomicUnit=on
  r_n : Outport
  h_n : Outport  Port=2
  wires:
  Constant1/1 -> MATLAB Function1/2(target)
  pos/1 -> MATLAB Function1/1(pos)
  Constant3/1 -> MATLAB Function1/4(r_max)
  MATLAB Function1/1(r_n) -> r_n/1
  MATLAB Function1/2(h_n) -> h_n/1
  Constant4/1 -> MATLAB Function1/5(h_min)
  Constant2/1 -> MATLAB Function1/3(r_min)
  Constant5/1 -> MATLAB Function1/6(h_max)

== system SAC_simulink/SIGNAL_PROCESSING /Observation vector costruction/Subsystem1 ==
  yaw : Inport
  Constant : Constant  Value=yaw_min
  Constant1 : Constant  Value=yaw_max
  MATLAB Function : MATLAB Function  TreatAsAtomicUnit=on
  yaw_n : Outport
  wires:
  Constant/1 -> MATLAB Function/2(yaw_min)
  Constant1/1 -> MATLAB Function/3(yaw_max)
  yaw/1 -> MATLAB Function/1(yaw)
  MATLAB Function/1(yaw_n) -> yaw_n/1

== system SAC_simulink/SIGNAL_PROCESSING /Observation vector costruction/Subsystem2 ==
  pos : Inport
  target : Inport  Port=2
  Constant : Constant  Value=r_min
  Constant1 : Constant  Value=r_max
  MATLAB Function2 : MATLAB Function  TreatAsAtomicUnit=on
  r_n : Outport
  wires:
  MATLAB Function2/1(r_n) -> r_n/1
  target/1 -> MATLAB Function2/2(target)
  pos/1 -> MATLAB Function2/1(pos)
  Constant1/1 -> MATLAB Function2/4(r_max)
  Constant/1 -> MATLAB Function2/3(r_min)

== system SAC_simulink/SIGNAL_PROCESSING /Observation vector costruction/Subsystem3 ==
  pos : Inport
  target : Inport  Port=2
  vel : Inport  Port=3
  MATLAB Function4 : MATLAB Function  TreatAsAtomicUnit=on
  angle_n : Outport
  wires:
  target/1 -> MATLAB Function4/2(target)
  vel/1 -> MATLAB Function4/3(vel)
  MATLAB Function4/1(angle_n) -> angle_n/1
  pos/1 -> MATLAB Function4/1(pos)

== system SAC_simulink/SIGNAL_PROCESSING /Observation vector costruction/Subsystem4 ==
  err_psi : Inport
  MATLAB Function : MATLAB Function  TreatAsAtomicUnit=on
  err_psi_norm : Outport
  wires:
  MATLAB Function/1(err_psi_norm) -> err_psi_norm/1
  err_psi/1 -> MATLAB Function/1(err_psi)

== system SAC_simulink/SIGNAL_PROCESSING /Observation vector costruction/Subsystem5 ==
  idx : Inport
  Multiply : Gain  Gain=1/ max_idx
  idx_n : Outport
  wires:
  idx/1 -> Multiply/1
  Multiply/1 -> idx_n/1

== system SAC_simulink/SIGNAL_PROCESSING /Observation vector costruction/Subsystem6 ==
  In1 : Inport
  Multiply : Gain  Gain=1/delta_a_max
  Out1 : Outport
  wires:
  In1/1 -> Multiply/1
  Multiply/1 -> Out1/1

== system SAC_simulink/SIGNAL_PROCESSING /Observation vector costruction/Subsystem7 ==
  action_prev : Inport
  Constant : Constant  Value=action_limits_upper
  Constant1 : Constant  Value=action_limits_lower
  MATLAB Function : MATLAB Function  TreatAsAtomicUnit=on
  action_prev_n : Outport
  wires:
  MATLAB Function/1(action_prev_n) -> action_prev_n/1
  action_prev/1 -> MATLAB Function/3(action_prev)
  Constant/1 -> MATLAB Function/1(action_limits_upper)
  Constant1/1 -> MATLAB Function/2(action_limits_lower)

== system SAC_simulink/SIGNAL_PROCESSING /Observation vector costruction/h_normalizzation ==
  h : Inport
  Constant1 : Constant  Value=h_min
  Constant2 : Constant  Value=h_max
  MATLAB Function : MATLAB Function  TreatAsAtomicUnit=on
  h_n : Outport
  wires:
  Constant2/1 -> MATLAB Function/3(h_max)
  Constant1/1 -> MATLAB Function/2(h_min)
  h/1 -> MATLAB Function/1(h)
  MATLAB Function/1(h_n) -> h_n/1

== system SAC_simulink/SIGNAL_PROCESSING /Reward_Assembly_SubSys/Reward_FlushFlag_Generator ==
  Clock : Clock
  Constant1 : Constant  Value=Ts
  Constant2 : Constant  Value=t_step
  MATLAB Function1 : MATLAB Function  TreatAsAtomicUnit=on
  Scope : Scope
      settings: ActiveDisplayYMinimum=-0.12499999999999997  ActiveDisplayYMaximum=1.125  DataLoggingVariableName=ScopeData20
  flush_flag : Outport
  wires:
  Constant1/1 -> MATLAB Function1/2(Ts)
  Constant2/1 -> MATLAB Function1/3(t_step)
  Clock/1 -> MATLAB Function1/1(t)
  MATLAB Function1/1(flush_flag) -> Scope/1, flush_flag/1

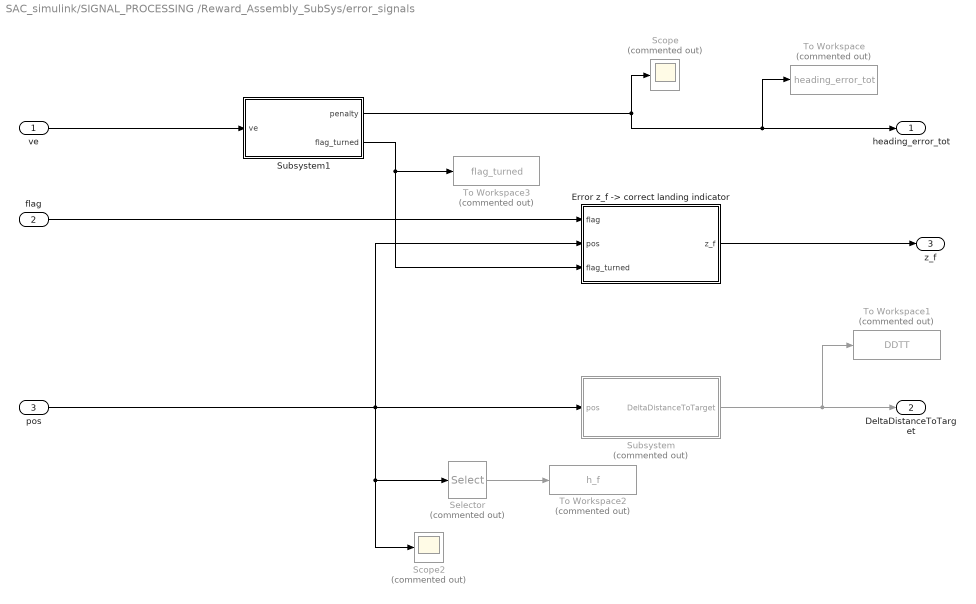
== system SAC_simulink/SIGNAL_PROCESSING /Reward_Assembly_SubSys/error_signals ==
  ve : Inport
  flag : Inport  Port=2
  pos : Inport  Port=3
  "Error z_f -> correct landing indicator" : Subsystem
  Scope : Scope  Commented=on
      settings: ActiveDisplayYMinimum=-6766.0396190901674  ActiveDisplayYMaximum=1554.08049498303  DataLoggingVariableName=ScopeData26
  Scope2 : Scope  Commented=on
      settings: ActiveDisplayYMinimum=-566.65982719608826  ActiveDisplayYMaximum=599.93844476479444  DataLoggingVariableName=ScopeData38
  Selector : Selector  Commented=on  InputPortWidth=3  IndexOptions=Index vector (dialog)  Indices=[3]  OutputSizes=1
  Subsystem : Subsystem  Commented=on
  Subsystem1 : Subsystem
  To Workspace : ToWorkspace  Commented=on  VariableName=heading_error_tot  SaveFormat=Timeseries  SampleTime=-1
  To Workspace1 : ToWorkspace  Commented=on  VariableName=DDTT  SaveFormat=Timeseries  SampleTime=-1
  To Workspace2 : ToWorkspace  Commented=on  VariableName=h_f  SaveFormat=Timeseries  SampleTime=-1
  To Workspace3 : ToWorkspace  Commented=on  VariableName=flag_turned  SaveFormat=Timeseries  SampleTime=-1
  heading_error_tot : Outport
  DeltaDistanceToTarget : Outport  Port=2
  z_f : Outport  Port=3
  wires:
  Subsystem1/1(penalty) -> To Workspace/1, heading_error_tot/1, Scope/1
  pos/1 -> "Error z_f -> correct landing indicator"/2(pos), Scope2/1, Selector/1, Subsystem/1(pos)
  ve/1 -> Subsystem1/1(ve)
  flag/1 -> "Error z_f -> correct landing indicator"/1(flag)
  "Error z_f -> correct landing indicator"/1(z_f) -> z_f/1
  Subsystem/1(DeltaDistanceToTarget) -> To Workspace1/1, DeltaDistanceToTarget/1
  Subsystem1/2(flag_turned) -> "Error z_f -> correct landing indicator"/3(flag_turned), To Workspace3/1
  Selector/1 -> To Workspace2/1

== system SAC_simulink/SIGNAL_PROCESSING /Reward_Assembly_SubSys/isFirstStep_Flag_Generator ==
  Constant1 : Constant  Value=0
  Memory1 : Memory  InitialCondition=1
  Out1 : Outport
  wires:
  Constant1/1 -> Memory1/1
  Memory1/1 -> Out1/1

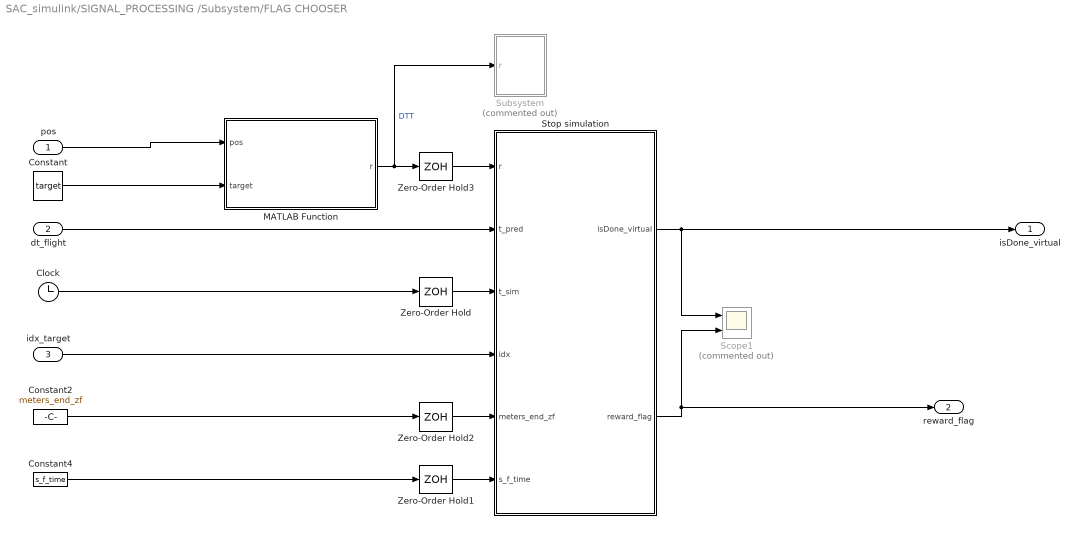
== system SAC_simulink/SIGNAL_PROCESSING /Subsystem/FLAG CHOOSER ==
  pos : Inport
  dt_flight : Inport  Port=2
  idx_target : Inport  Port=3
  Clock : Clock
  Constant : Constant  Value=target
  Constant2 : Constant  Value=meters_end_zf
  Constant4 : Constant  Value=s_f_time
  MATLAB Function : MATLAB Function  TreatAsAtomicUnit=on
  Scope1 : Scope  Commented=on  NumInputPorts=2
      settings: ActiveDisplayYMinimum=-1.375  ActiveDisplayYMaximum=2.375  DataLoggingVariableName=ScopeData31
  Stop simulation : MATLAB Function  TreatAsAtomicUnit=on
  Subsystem : Subsystem  Commented=on
  Zero-Order Hold{,1..3} (4 alike) : ZeroOrderHold  SampleTime=-1
  isDone_virtual : Outport
  reward_flag : Outport  Port=2
  wires:
  Constant2/1 -> Zero-Order Hold2/1
  Constant/1 -> MATLAB Function/2(target)
  Constant4/1 -> Zero-Order Hold1/1
  idx_target/1 -> Stop simulation/4(idx)
  pos/1 -> MATLAB Function/1(pos)
  dt_flight/1 -> Stop simulation/2(t_pred)
  Clock/1 -> Zero-Order Hold/1
  Stop simulation/2(reward_flag) -> Scope1/2, reward_flag/1
  MATLAB Function/1(r) -> Subsystem/1(r), Zero-Order Hold3/1  "DTT"
  Stop simulation/1(isDone_virtual) -> isDone_virtual/1, Scope1/1
  Zero-Order Hold/1 -> Stop simulation/3(t_sim)
  Zero-Order Hold2/1 -> Stop simulation/5(meters_end_zf)
  Zero-Order Hold1/1 -> Stop simulation/6(s_f_time)
  Zero-Order Hold3/1 -> Stop simulation/1(r)

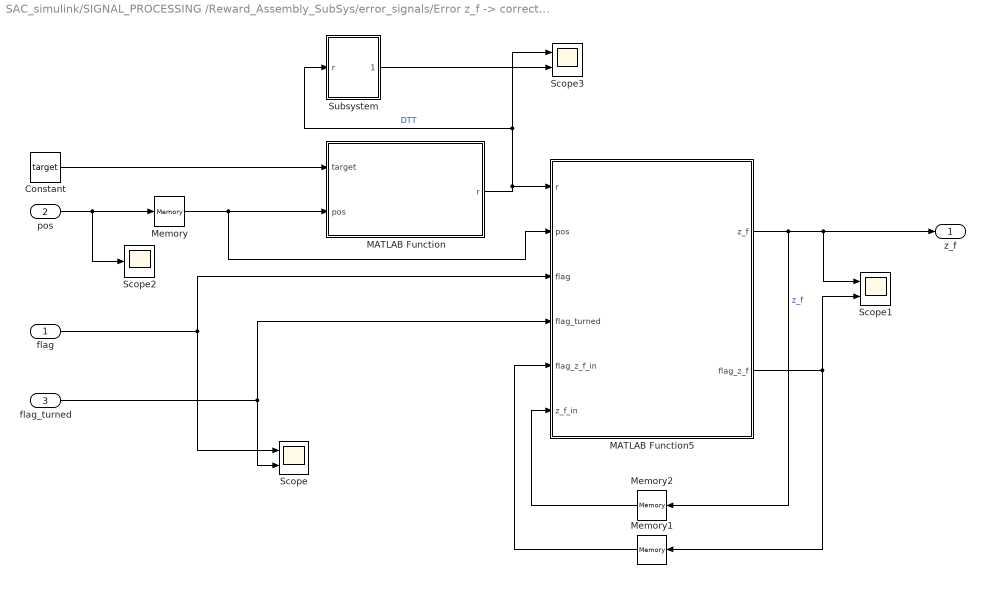
== system SAC_simulink/SIGNAL_PROCESSING /Reward_Assembly_SubSys/error_signals/Error z_f -> correct landing indicator ==
  flag : Inport
  pos : Inport  Port=2
  flag_turned : Inport  Port=3
  Constant : Constant  Value=target
  MATLAB Function : MATLAB Function  TreatAsAtomicUnit=on
  MATLAB Function5 : MATLAB Function  TreatAsAtomicUnit=on
  Memory : Memory  InitialCondition=X0
  Memory1 : Memory
  Memory2 : Memory
  Scope : Scope  NumInputPorts=2
      settings: ActiveDisplayYMinimum=-0.24999999999999994  ActiveDisplayYMaximum=2.25  DataLoggingVariableName=ScopeData11
  Scope1 : Scope  NumInputPorts=2
      settings: ActiveDisplayYMinimum=-0.12499999999999997  ActiveDisplayYMaximum=1.125  DataLoggingVariableName=ScopeData39
  Scope2 : Scope
      settings: ActiveDisplayYMinimum=-791.10194314840271  ActiveDisplayYMaximum=619.91748833562463  DataLoggingVariableName=ScopeData40
  Scope3 : Scope  NumInputPorts=2
      settings: ActiveDisplayYMinimum=-81.249999999999986  ActiveDisplayYMaximum=731.25  DataLoggingVariableName=ScopeData41
  Subsystem : Subsystem
  z_f : Outport
  wires:
  flag/1 -> Scope/1, MATLAB Function5/3(flag)
  flag_turned/1 -> Scope/2, MATLAB Function5/4(flag_turned)
  Memory/1 -> MATLAB Function5/2(pos), MATLAB Function/2(pos)
  Constant/1 -> MATLAB Function/1(target)
  pos/1 -> Scope2/1, Memory/1
  MATLAB Function5/1(z_f) -> Memory2/1, z_f/1, Scope1/1  "z_f"
  MATLAB Function/1(r) -> Subsystem/1(r), Scope3/1, MATLAB Function5/1(r)  "DTT"
  Subsystem/1(r_less_15) -> Scope3/2
  MATLAB Function5/2(flag_z_f) -> Scope1/2, Memory1/1
  Memory1/1 -> MATLAB Function5/5(flag_z_f_in)
  Memory2/1 -> MATLAB Function5/6(z_f_in)

== system SAC_simulink/SIGNAL_PROCESSING /Reward_Assembly_SubSys/error_signals/Subsystem ==
  pos : Inport
  Constant : Constant  Value=target
  Constant1 : Constant  Value=0
  MATLAB Function1 : MATLAB Function  TreatAsAtomicUnit=on
  Memory : Memory
  Memory1 : Memory  InitialCondition=1
  DeltaDistanceToTarget : Outport
  wires:
  Constant/1 -> MATLAB Function1/2(target)  "target"
  MATLAB Function1/1(DeltaDistanceToTarget) -> DeltaDistanceToTarget/1
  Constant1/1 -> Memory1/1
  Memory1/1 -> MATLAB Function1/3(isFirstStep)
  pos/1 -> MATLAB Function1/1(pos)
  MATLAB Function1/2(r_prev) -> Memory/1
  Memory/1 -> MATLAB Function1/4("r_prev ")

== system SAC_simulink/SIGNAL_PROCESSING /Reward_Assembly_SubSys/error_signals/Subsystem1 ==
  ve : Inport
  Clock : Clock
  MATLAB Function : MATLAB Function  TreatAsAtomicUnit=on
  MATLAB Function1 : MATLAB Function  Commented=on  TreatAsAtomicUnit=on
  Memory1 : Memory  Commented=on
  Scope : Scope
      settings: ActiveDisplayYMinimum=-0.020367860036501595  ActiveDisplayYMaximum=1.0127132074359313  DataLoggingVariableName=ScopeData27
  To Workspace10 : ToWorkspace  Commented=on  VariableName=heading_error_tot  SaveFormat=Timeseries  SampleTime=-1
      settings: MaxDataPoints=1
  Zero-Order Hold : ZeroOrderHold  SampleTime=-1
  penalty : Outport
  flag_turned : Outport  Port=2
  wires:
  MATLAB Function1/1(heading_error) -> To Workspace10/1
  Memory1/1 -> MATLAB Function1/1(err_psi)
  ve/1 -> MATLAB Function/1(ve)
  MATLAB Function/1(penalty) -> penalty/1
  MATLAB Function/2(has_spun) -> Scope/1, flag_turned/1
  Clock/1 -> Zero-Order Hold/1
  Zero-Order Hold/1 -> MATLAB Function/2(current_time)

== system SAC_simulink/SIGNAL_PROCESSING /Subsystem/FLAG CHOOSER/Subsystem ==
  r : Inport
  Constant : Constant
  Constant1 : Constant  Value=0
  Stop Simulation : Stop
  Switch : Switch  Threshold=15  SaturateOnIntegerOverflow=off  InputSameDT=off
  wires:
  Switch/1 -> Stop Simulation/1
  Constant1/1 -> Switch/1
  Constant/1 -> Switch/3
  r/1 -> Switch/2

== system SAC_simulink/SIGNAL_PROCESSING /Reward_Assembly_SubSys/error_signals/Error z_f -> correct landing indicator/Subsystem ==
  r : Inport
  Constant : Constant
  Constant1 : Constant  Value=0
  Switch : Switch  Threshold=15  SaturateOnIntegerOverflow=off  InputSameDT=off
  r_less_15 : Outport
  wires:
  Switch/1 -> r_less_15/1
  Constant1/1 -> Switch/1
  Constant/1 -> Switch/3
  r/1 -> Switch/2

== matlab function SAC_simulink/SIGNAL_PROCESSING /Observation vector costruction/Subsystem3/MATLAB Function4 ==
  data: pos input; target input; angle_n output; vel input
function angle_n = fun_angle_n(pos, target, vel)
    % 1. Vettore dalla posizione al target
    r = target(1:2) - pos(1:2);
    
    % 2. Normalizzazione vettori 
    r_u = r / norm(r);
    v_u = vel(1:2) / norm(vel);
    
    % 3. Calcolo dell'angolo con segno usando atan2
    % atan2(y, x) restituisce l'angolo tra [-pi, pi]
    % Usiamo il determinante (cross product 2D) e il prodotto scalare
    angle_rad = atan2(v_u(1)*r_u(2) - v_u(2)*r_u(1), dot(v_u, r_u));
    
    % 4. Normalizzazione nell'intervallo [-1, 1]
    angle_n = angle_rad / pi;
end

== matlab function SAC_simulink/SIGNAL_PROCESSING /Subsystem/FLAG CHOOSER/Stop simulation ==
  data: r input; isDone_virtual output; t_pred input; t_sim input; idx input; meters_end_zf input; s_f_time input; reward_flag output
function [isDone_virtual, reward_flag] = radius_comp(r, t_pred, t_sim, idx, meters_end_zf, s_f_time)
    
    % Dichiara una variabile che mantiene il suo valore tra le chiamate
    persistent has_finished;
    
    % Inizializza la variabile solo la primissima volta che chiami la funzione
    if isempty(has_finished)
        has_finished = false;
    end

    % La tua logica originale
    if idx >= 199.5 && r <= meters_end_zf
        reward_flag = 1;
        temp_done = 1;
    elseif idx >= 199.5 && t_pred * s_f_time <= t_sim
        reward_flag = 2;
        temp_done = 1;
    elseif t_pred * s_f_time < t_sim
        reward_flag = 3;
        temp_done = 1;
    else
        reward_flag = 0; 
        temp_done = 0;
    end
    
    % Se è diventato 1 in questo step, salvalo in modo permanente
    if temp_done == 1
        has_finished = true;
    end
    
    % Assegna l'output finale: se ha mai raggiunto l'1, sarà sempre 1
    if has_finished
        isDone_virtual = 1;
    else
        isDone_virtual = temp_done;
    end
end

== matlab function SAC_simulink/SIGNAL_PROCESSING /Subsystem/FLAG CHOOSER/MATLAB Function ==
  data: pos input; r output; target input
function r = radius_pos2target(pos, target)
r = sqrt((pos(1)-target(1))^2 + (pos(2)-target(2))^2);
end

== matlab function SAC_simulink/SIGNAL_PROCESSING /Observation vector costruction/Subsystem7/MATLAB Function ==
  data: action_prev_n output; action_limits_upper input; action_limits_lower input; action_prev input
function action_prev_n = fcn(action_limits_upper, action_limits_lower, action_prev)
    % Normalizzazione Min-Max tra 0 e 1
    action_prev_n = (action_prev - action_limits_lower) ./ (action_limits_upper - action_limits_lower);
end

== matlab function SAC_simulink/SIGNAL_PROCESSING /Reward_Assembly_SubSys/error_signals/Subsystem1/MATLAB Function ==
  data: ve input; penalty output; current_time input; has_spun output
function [penalty, has_spun] = velocity_window_penalty(ve, current_time)
    % persistent per il Ring Buffer
    persistent buffer_theta
    persistent idx
    persistent last_time
    persistent buffer_full
    
    barrier = 12.5; % [s]
    sampling = 0.25; % [s]

    N = barrier / sampling; 
    
    vx = ve(1);
    vy = ve(2);
    
    % Inizializzazione al primo step
    if isempty(buffer_theta)
        buffer_theta = zeros(1, N);
        idx = 1;
        last_time = -0.25;  
        buffer_full = false;
    end
    
    % Valori di default in uscita se tutto va bene
    penalty = 0;
    has_spun = 0;
    
    % 1. Calcolo angolo attuale (salvato in radianti per una matematica più sicura)
    theta_current = atan2(vy, vx); 
    
    % 2. Controlliamo se sono passati almeno 0.25 secondi dall'ultimo salvataggio
    if (current_time - last_time) >= 0.25
        
        if buffer_full
            theta_old = buffer_theta(idx);
            
            % Calcolo differenza angolare pulita (normalizzata tra -pi e pi)
            % Questo evita bug se il drone passa dal nord (es. da +179 a -179 gradi)
            delta_rad = theta_current - theta_old;
            delta_rad = atan2(sin(delta_rad), cos(delta_rad)); 
            
            % Convertiamo in gradi solo alla fine per fare il controllo
            delta_deg = abs(delta_rad * 180 / pi);
            
            % Controllo Soglia: Più di 120 gradi in 20 secondi
            if delta_deg > 120
                % ATTIVA LO SCALINO
                penalty = -500; 
                has_spun = 1;
                
                % --- IL TRUCCO DEL RESET ---
                % Svuotiamo la memoria e facciamo ripartire l'analisi da zero.
                % Questo distrugge il "muro rosso" del grafico: per i prossimi 20
                % secondi il buffer_full sarà false e non scatteranno altre penalità.
                buffer_full = false;
                idx = 1;
                
                % Salviamo il valore attuale come "nuovo punto zero" e usciamo
                buffer_theta(idx) = theta_current;
                last_time = current_time;
                return; % Blocca l'esecuzione qui per questo step
            end
        end
        
        % Se non c'è stata nessuna penalità estrema, procediamo col salvataggio normale
        buffer_theta(idx) = theta_current;
        last_time = current_time;
        
        % Avanza il puntatore (se supera 80, torna a 1 e segna il buffer come pieno)
        idx = idx + 1;
        if idx > N
            idx = 1;
            buffer_full = true; 
        end
    end
    
    % NOTA SUL -250 OGNI 0.25s: 
    % Se vuoi che mentre il buffer si riempie normalmente l'agente riceva 
    % un malus costante di -250 ad ogni step di 0.25s, ti basta aggiungere:
    % penalty = penalty - 250; 
    % qui alla fine, prima dell'end della funzione. Ma fai attenzione: un malus
    % costante di -250 ogni 0.25s significa -1000 punti al secondo in volo libero!
end
